simulink model "RRT_guidance"  (R2025b)
settings: Solver=VariableStepAuto  StartTime=0.0  StopTime=14.29  RelTol=1e-3
values from neighbouring files (symbols this model uses):
  waypoints_RRT_smoothed = [pthSmoothed1.States(:,1), pthSmoothed1.States(:,2), pthSmoothed1.States(:,3)]    [Path_finding.m]
libraries: uavalgslib x2
settings DataIOCC: ReturnWorkspaceOutputs=off

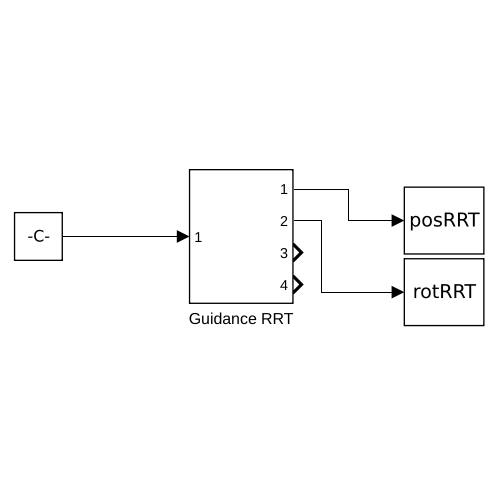
[thumbnail: Simulink's stored preview of the top-level diagram]
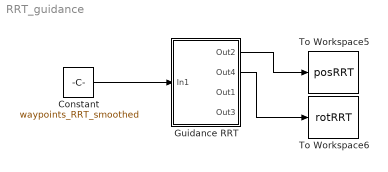
== system RRT_guidance ==
  Constant : Constant  Value=waypoints_RRT_smoothed
  Guidance RRT : Subsystem
  To Workspace5 : ToWorkspace  VariableName=posRRT  SampleTime=-1
      settings: Save2DSignal=2-D array (concatenate along first dimension)
  To Workspace6 : ToWorkspace  VariableName=rotRRT  SampleTime=-1
      settings: Save2DSignal=2-D array (concatenate along first dimension)
  wires:
  Constant/1 -> Guidance RRT/1(In1)
  Guidance RRT/1(Out2) -> To Workspace5/1
  Guidance RRT/2(Out4) -> To Workspace6/1

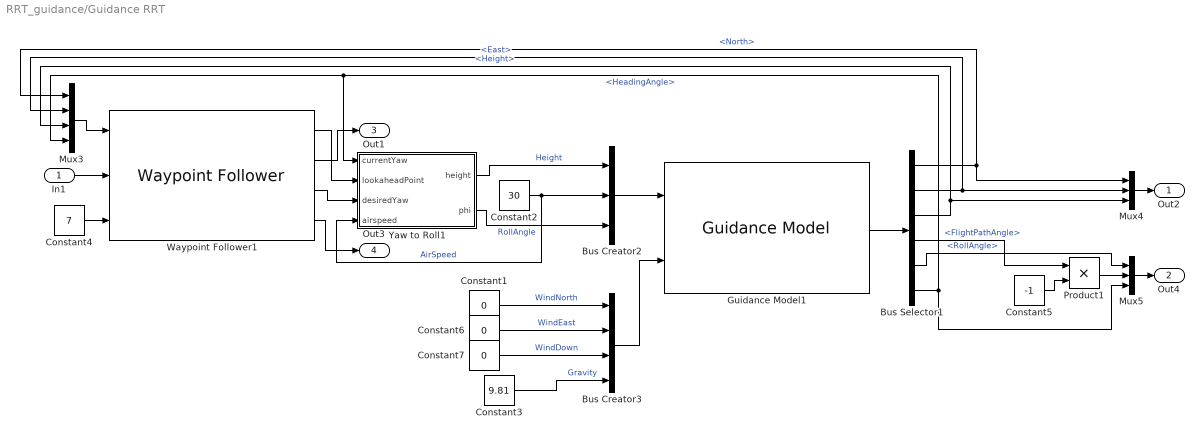
== system RRT_guidance/Guidance RRT ==
  In1 : Inport
  Bus Creator2 : BusCreator  Inputs=3  OutDataTypeStr=Bus: FixedWingGuidanceControlBus  NonVirtualBus=on
  Bus Creator3 : BusCreator  Inputs=4  OutDataTypeStr=Bus: FixedWingGuidanceEnvironmentBus  NonVirtualBus=on
  Bus Selector1 : BusSelector  OutputSignals=North,East,Height,FlightPathAngle,RollAngle,HeadingAngle
  Constant1 : Constant  Value=0
  Constant2 : Constant  Value=30
  Constant3 : Constant  Value=9.81
  Constant4 : Constant  Value=7
  Constant5 : Constant  Value=-1
  Constant6 : Constant  Value=0
  Constant7 : Constant  Value=0
  Guidance Model1 : uavalgslib/Guidance Model  ModelType=FixedWingGuidance  NumInstances=1  SpecifiedDataType=double  SimulateUsing=Interpreted execution  InitialWorldPositionMultirotor=[0; 0; 0]  InitialWorldVelocityMultirotor=[0; 0; 0]  InitialEulerZYXMultirotor=[0; 0; 0]  InitialBodyAngularRateRPYMultirotor=[0; 0; 0]  InitialThrustMultirotor=0  InitialNorthFixedWing=0  InitialEastFixedWing=0  InitialHeightFixedWing=50  InitialAirSpeedFixedWing=30  InitialHeadingAngleFixedWing=0  InitialFlightPathAngleFixedWing=0  InitialRollAngleFixedWing=0  InitialRollAngleRateFixedWing=0  PDRollMultirotor=[3402.97,116.67]  PDPitchMultirotor=[3402.97, 116.67]  PYawRateMultirotor=1950  PThrustMultirotor=3900  MassMultirotor=0.1  PHeightFixedWing=3.9  PHeadingAngleFixedWing=3.9  PFlightPathAngleFixedWing=39  PDRollFixedWing=[3402.97, 116.67]  PAirSpeedFixedWing=1  FlightPathAngleLimitsFixedWing=[-pi/2, pi/2]  StateBusName='FixedWingGuidanceStateBus'  ControlBusName='FixedWingGuidanceControlBus'  EnvironmentBusName='FixedWingGuidanceEnvironmentBus'  DataType=double
  Mux3 : Mux
  Mux4 : Mux  Inputs=3
  Mux5 : Mux  Inputs=3
  Product1 : Product
  Waypoint Follower1 : uavalgslib/Waypoint Follower  UAVType=fixed-wing  StartFrom=first  TransitionRadiusSource=internal  TransitionRadius=10  MinLookaheadDistance=0.1  HoverAtLastWaypoint=off  YawInput=off  ShowCrossTrackErrorOutput=off  ShowStatusOutput=off  SimulateUsing=Interpreted execution
  Yaw to Roll1 : MATLAB Function  TreatAsAtomicUnit=on
  Out2 : Outport
  Out4 : Outport  Port=2
  Out1 : Outport  Port=3
  Out3 : Outport  Port=4
  wires:
  Bus Creator2/1 -> Guidance Model1/1
  Mux4/1 -> Out2/1
  Waypoint Follower1/4 -> Out3/1
  Waypoint Follower1/3 -> Yaw to Roll1/3(desiredYaw)
  Bus Creator3/1 -> Guidance Model1/2
  Yaw to Roll1/2(phi) -> Bus Creator2/3  "RollAngle"
  Mux3/1 -> Waypoint Follower1/1
  Constant3/1 -> Bus Creator3/4  "Gravity"
  Waypoint Follower1/1 -> Yaw to Roll1/2(lookaheadPoint)
  Yaw to Roll1/1(height) -> Bus Creator2/1  "Height"
  Waypoint Follower1/2 -> Out1/1
  Guidance Model1/1 -> Bus Selector1/1
  Constant1/1 -> Bus Creator3/1  "WindNorth"
  Bus Selector1/2 -> Mux4/2, Mux3/2  "<East>"
  Bus Selector1/1 -> Mux3/1, Mux4/1  "<North>"
  Bus Selector1/3 -> Mux3/3, Mux4/3  "<Height>"
  Constant7/1 -> Bus Creator3/3  "WindDown"
  Constant6/1 -> Bus Creator3/2  "WindEast"
  Bus Selector1/4 -> Product1/1  "<FlightPathAngle>"
  Product1/1 -> Mux5/2
  Constant5/1 -> Product1/2
  Mux5/1 -> Out4/1
  In1/1 -> Waypoint Follower1/2
  Constant4/1 -> Waypoint Follower1/3
  Constant2/1 -> Yaw to Roll1/4(airspeed), Bus Creator2/2  "AirSpeed"
  Bus Selector1/6 -> Mux3/4, Yaw to Roll1/1(currentYaw), Mux5/3  "<HeadingAngle>"
  Bus Selector1/5 -> Mux5/1  "<RollAngle>"

== matlab function RRT_guidance/Guidance RRT/Yaw to Roll1 ==
  data: currentYaw input; lookaheadPoint input; height output; desiredYaw input; phi output; airspeed input
function [height, phi]= yawToRoll(currentYaw, lookaheadPoint, desiredYaw, airspeed)
% Convert desired yaw rate into coordinated turn roll angle
g = 9.81;
dt = 0.05;
yawRate = wrapToPi(desiredYaw - currentYaw) / dt;

phi = atan((airspeed * yawRate) / g);

height = lookaheadPoint(3);
end
